simulink model "TCS0731"  (R2022b)
settings: Solver=VariableStepAuto  StartTime=0.0  StopTime=30  FixedStep=0.01  RelTol=1e-3
libraries: simulink x8, Solver_SF x1
settings Model: Creator=12045  LastModifiedBy=12045
settings DebuggingCC: ParameterPrecisionLossMsg=none

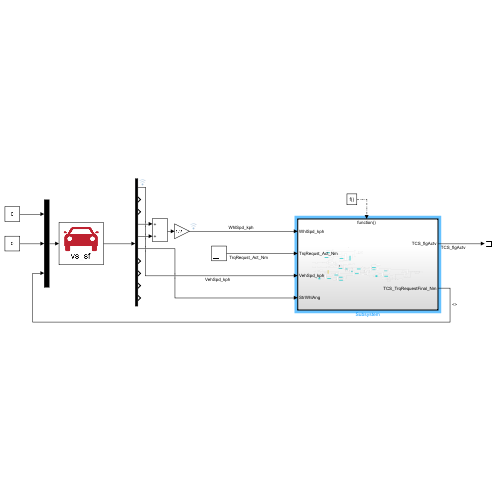
[thumbnail: Simulink's stored preview of the top-level diagram]
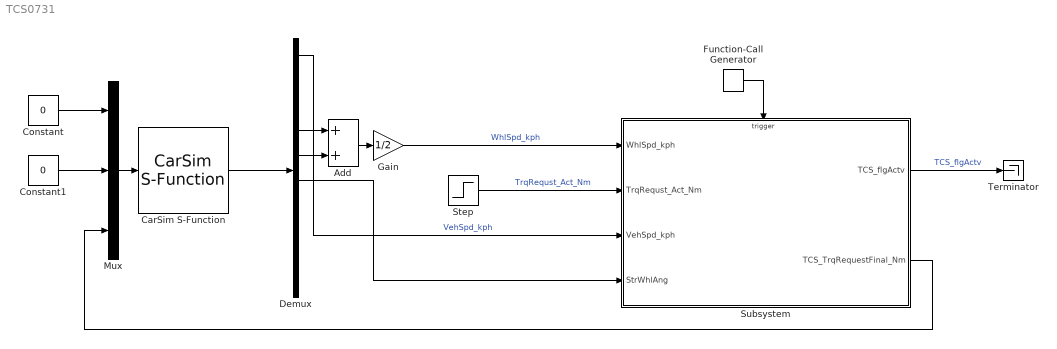
== system TCS0731 ==
  Add : Sum
  CarSim S-Function : Solver_SF/CarSim S-Function  Priority=1  SIMFILE=simfile.sim  Run_RTs=off  vs_state_ind=Run  StopMode_ind=Vehicle Model
  Constant : Constant  Value=0
  Constant1 : Constant  Value=0
  Demux : Demux  Outputs=10
  Function-Call Generator : simulink/Ports & Subsystems/Function-Call Generator  sample_time=0.01  numberOfIterations=1  DisallowWideOutput=off
  Gain : Gain  Gain=1/2
  Mux : Mux  Inputs=3
  Step : Step  After=80  SampleTime=0
  Subsystem : Subsystem
  Terminator : Terminator
  wires:
  Subsystem/1(TCS_flgActv) -> Terminator/1  "TCS_flgActv"
  Subsystem/2(TCS_TrqRequestFinal_Nm) -> Mux/3
  Function-Call Generator/1 -> Subsystem/Trigger
  Gain/1 -> Subsystem/1(WhlSpd_kph)  "WhlSpd_kph"
  Step/1 -> Subsystem/2(TrqRequst_Act_Nm)  "TrqRequst_Act_Nm"
  Demux/1 -> Subsystem/3(VehSpd_kph)  "VehSpd_kph"
  Mux/1 -> CarSim S-Function/1
  Constant/1 -> Mux/1
  Constant1/1 -> Mux/2
  CarSim S-Function/1 -> Demux/1
  Demux/4 -> Add/1
  Demux/5 -> Add/2
  Add/1 -> Gain/1
  Demux/6 -> Subsystem/4(StrWhlAng)

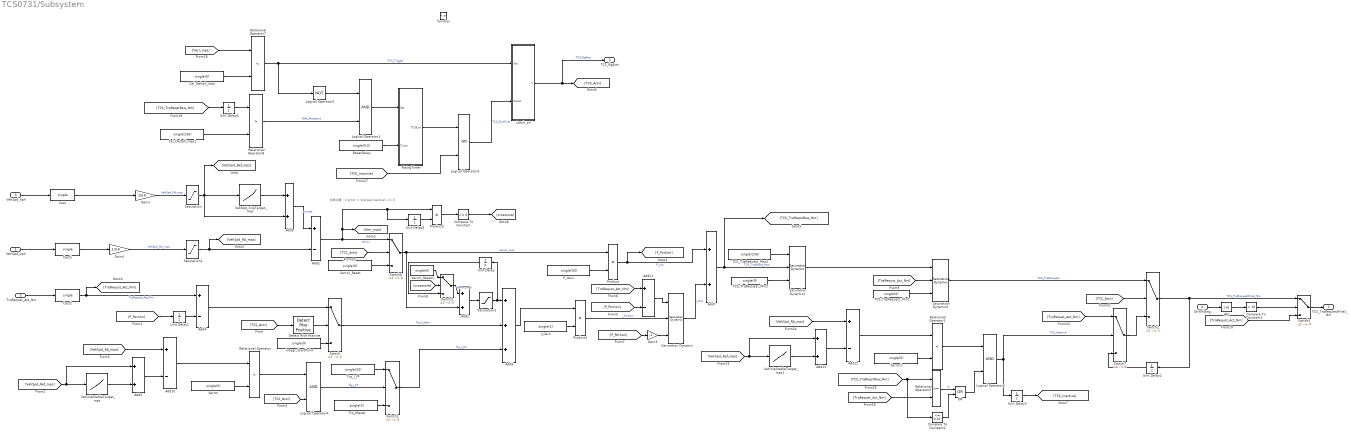
== system TCS0731/Subsystem ==
  note: 特殊设置：V error = Vtarget-Vactual <= 0
  WhlSpd_kph : Inport
  TrqRequst_Act_Nm : Inport  Port=2
  VehSpd_kph : Inport  Port=3
  StrWhlAng : Inport  Port=4
  function : TriggerPort  TriggerType=function-call  VariantControl=(inherit)
  Abs : Abs  SaturateOnIntegerOverflow=off
  Add{1,4,10..12} (5 alike) : Sum  Inputs=+-
  Add{2,5,7,9,13} (5 alike) : Sum
  Add6 : Sum  Inputs=+++
  Cal_DeltaV_mps : Constant  Value=single(0)
  Cal_DeltaV_mps1 : Constant  Value=single(235)
  Cast : DataTypeConversion  OutDataTypeStr=single  SaturateOnIntegerOverflow=off  RndMeth=Floor
  Cast1 : DataTypeConversion  OutDataTypeStr=single  SaturateOnIntegerOverflow=off  RndMeth=Floor
  Cast2 : DataTypeConversion  OutDataTypeStr=single  SaturateOnIntegerOverflow=off  RndMeth=Floor
  Compare To Constant : simulink/Logic and Bit Operations/Compare To Constant  relop=<=  const=0  OutDataTypeStr=boolean
  Compare To Constant1 : simulink/Logic and Bit Operations/Compare To Constant  relop=<  const=10  OutDataTypeStr=boolean
  Compare To Constant2 : simulink/Logic and Bit Operations/Compare To Constant  relop=<=  const=0.01  OutDataTypeStr=boolean
  Detect Rise Positive : simulink/Logic and Bit Operations/Detect Rise Positive  vinit=0  OutDataTypeStr=boolean
  Gain1 : Gain  Gain=1/3.6
  Gain3 : Gain  Gain=-1
  Gain4 : Gain  Gain=1/3.6
  I_Gain : Constant  Value=single(2)
  Integr_StartPoint : Constant  Value=single(0)
  Latch_on : Subsystem
  Logical Operator1 : Logic  AllPortsSameDT=off  OutDataTypeStr=boolean
  Logical Operator2 : Logic  Operator=NOT  AllPortsSameDT=off  OutDataTypeStr=boolean
  Logical Operator3 : Logic  Operator=OR  AllPortsSameDT=off  OutDataTypeStr=boolean
  Logical Operator4 : Logic  AllPortsSameDT=off  OutDataTypeStr=boolean
  Logical Operator5 : Logic  AllPortsSameDT=off  OutDataTypeStr=boolean
  OR : Logic  Operator=OR  AllPortsSameDT=off  OutDataTypeStr=boolean
  P_Gain : Constant  Value=single(20)
  Product : Product
  Product1 : Product
  Product2 : Product
  Relational Operator : RelationalOperator  Operator=<  OutDataTypeStr=boolean  RndMeth=Simplest  InputSameDT=off
  Relational Operator1 : RelationalOperator  Operator=<  OutDataTypeStr=boolean  RndMeth=Simplest  InputSameDT=off
  Relational Operator2 : RelationalOperator  OutDataTypeStr=boolean  RndMeth=Simplest  InputSameDT=off
  Relational Operator7 : RelationalOperator  Operator=<  OutDataTypeStr=boolean  RndMeth=Simplest  InputSameDT=off
  Relational Operator8 : RelationalOperator  Operator=>  OutDataTypeStr=boolean  RndMeth=Simplest  InputSameDT=off
  ResetDelay : Constant  Value=single(0.5)
  RisingTimer : Subsystem
  Saturation : Saturate  UpperLimit=40  LowerLimit=0
  Saturation Dynamic : simulink/Discontinuities/Saturation Dynamic  OutMin=[]  OutMax=[]  OutDataTypeStr=Inherit: Same as second input  OutDataType=fixdt(1, 16)  OutScaling=2^-10  DoSatur=off
  Saturation Dynamic1 : simulink/Discontinuities/Saturation Dynamic  OutMin=[]  OutMax=[]  OutDataTypeStr=Inherit: Same as second input  OutDataType=fixdt(1, 16)  OutScaling=2^-10  DoSatur=off
  Saturation Dynamic2 : simulink/Discontinuities/Saturation Dynamic  OutMin=[]  OutMax=[]  OutDataTypeStr=Inherit: Same as second input  OutDataType=fixdt(1, 16)  OutScaling=2^-10  DoSatur=off
  Saturation1 : Saturate  UpperLimit=50  LowerLimit=0
  Saturation2 : Saturate  UpperLimit=400  LowerLimit=-100
  Switch{,1..3,5..7} (7 alike) : Switch  Criteria=u2 ~= 0  SaturateOnIntegerOverflow=off  InputSameDT=off
  TCS_TrqRequest_Max2 : Constant  Value=single(235)
  TCS_TrqRequest_Min1 : Constant  Value=single(0)
  TCS_TrqRequest_Min2 : Constant  Value=single(0)
  Trq_IReset : Constant  Value=single(0)
  Trq_I_FF : Constant  Value=single(20)
  Unit Delay{,1..5} (6 alike) : UnitDelay  SampleTime=-1  HasFrameUpgradeWarning=on
  VehSpd_SlipTarget_mps : Lookup_n-D  NumberOfTableDimensions=1  BreakpointsForDimension1=[0 3 25 30]  Table=[0.3,0.3,2.5,2.5]  ExtrapMethod=Clip  InternalRulePriority=Speed  RndMeth=Simplest
  VehicleStableTarget_mps : Lookup_n-D  NumberOfTableDimensions=1  BreakpointsForDimension1=[0,3,25,30]  Table=[0.4,0.4,1.2,1.2]  ExtrapMethod=Clip  InternalRulePriority=Speed  RndMeth=Simplest
  VehicleStableTarget_mps1 : Lookup_n-D  NumberOfTableDimensions=1  BreakpointsForDimension1=[0,3,25,30]  Table=[0.2,0.2,1.2,1.2]  ExtrapMethod=Clip  InternalRulePriority=Speed  RndMeth=Simplest
  Verror : Constant  Value=single(0)
  Verror1 : Constant  Value=single(0)
  Verror_Reset : Constant  Value=single(0)
  Verror_Reset1 : Constant  Value=single(0)
  TCS_flgActv : Outport
  TCS_TrqRequestFinal_Nm : Outport  Port=2
  wires:
  TCS_TrqRequest_Max2/1 -> Saturation Dynamic1/1
  [TCS_Actv] -> Switch2/2
  [TrqRequst_Act_Nm] -> Switch7/1
  [VehSpd_Ref_mps] -> VehicleStableTarget_mps1/1, Add13/1
  Integr_StartPoint/1 -> Switch/3
  VehicleStableTarget_mps1/1 -> Add13/2
  [VehSpd_Ref_mps] -> Add5/1, VehicleStableTarget_mps/1
  [VehSpd_RA_mps] -> Add12/1
  [TCS_Actv] -> Switch6/2
  Gain4/1 -> Saturation1/1  "VehSpd_RA_mps"
  [TCS_Actv] -> Detect Rise Positive/1
  Saturation Dynamic1/1 -> Saturation Dynamic2/1
  Logical Operator3/1 -> Latch_on/2(Reset)  "TCS_ExitFinal"
  ResetDelay/1 -> RisingTimer/2(Timer)
  Latch_on/1(flg_TCSActv) -> TCS_flgActv/1, [TCS_Actv]  "TCS_flgActv"
  Unit Delay4/1 -> Relational Operator8/1
  WhlSpd_kph/1 -> Cast1/1
  Relational Operator1/1 -> Logical Operator5/1
  Product/1 -> [P_Portion], Add7/1  "P_out"
  Relational Operator7/1 -> Latch_on/1(Set), Logical Operator2/1  "TCS_Trigger"
  Switch/1 -> Add6/2  "Trq_I_Start"
  Trq_I_FF/1 -> Switch1/1
  Add13/1 -> Add12/2
  [TrqRequst_Act_Nm] -> Relational Operator2/2
  Add2/1 -> Saturation2/1
  TCS_TrqRequest_Min2/1 -> Saturation Dynamic1/3
  Add4/1 -> Switch/1
  [TCS_Inactive] -> Logical Operator3/2
  Add10/1 -> Relational Operator/1
  VehicleStableTarget_mps/1 -> Add5/2
  TrqRequst_Act_Nm/1 -> Cast2/1
  [P_Portion] -> Gain3/1
  Gain1/1 -> Saturation/1  "VehSpd_FA_mps"
  Saturation1/1 -> Add1/2, [VehSpd_RA_mps]
  Product1/1 -> Saturation Dynamic/2  "I_Portion"
  Logical Operator5/1 -> Unit Delay3/1, Switch7/2  "TCS_Inactive"
  Cal_DeltaV_mps1/1 -> Relational Operator8/2
  Add11/1 -> Saturation Dynamic/1
  Unit Delay3/1 -> [TCS_Inactive]
  Logical Operator1/1 -> RisingTimer/1(Set)
  [P_Portion] -> Add11/2
  Switch2/1 -> Switch5/1, Unit Delay2/1  "TCS_TrqRequestFinal_Nm"
  [TCS_TrqReqstRaw_Nm] -> Compare To Constant2/1, Relational Operator2/1
  Switch1/1 -> Add6/3  "Trq_I_FF"
  [VehSpd_RA_mps] -> Add10/1
  Unit Delay/1 -> Switch3/3
  Logical Operator2/1 -> Logical Operator1/1
  Trq_IReset/1 -> Switch1/3
  Verror1/1 -> Relational Operator1/2
  Relational Operator2/1 -> OR/1  "a"
  Switch7/1 -> Switch2/3
  Add12/1 -> Relational Operator1/1
  [P_Portion] -> Unit Delay1/1
  Unit Delay1/1 -> Add4/2
  Verror/1 -> Relational Operator/2
  Saturation Dynamic2/1 -> Switch2/1  "TCS_TrqRequest"
  [TrqRequst_Act_Nm] -> Saturation Dynamic2/2
  [TrqRequst_Act_Nm] -> Add11/1
  I_Gain/1 -> Product1/2
  Switch6/1 -> Product/1, Add2/2  "Verror_mps"
  Add9/1 -> Add1/1  "whlref"
  VehSpd_SlipTarget_mps/1 -> Add9/1
  [TCS_TrqReqstRaw_Nm] -> Unit Delay4/1
  Add5/1 -> Add10/2
  Saturation2/1 -> Unit Delay/1, Add6/1
  Add1/1 -> Switch6/1, [Verr_mps], Unit Delay5/1, Product2/1  "Verror"
  Verror_Reset/1 -> Switch6/3
  TCS_TrqRequest_Min1/1 -> Saturation Dynamic2/3
  Add7/1 -> Saturation Dynamic1/2, [TCS_TrqReqstRaw_Nm]  "TCS_TrqReqst_Raw"
  [Verr_mps] -> Relational Operator7/1
  Cal_DeltaV_mps/1 -> Relational Operator7/2
  Add6/1 -> Product1/1
  Relational Operator8/1 -> Logical Operator1/2  "fSat_Actuators"
  Relational Operator/1 -> Logical Operator4/1
  Saturation/1 -> Add9/2, VehSpd_SlipTarget_mps/1, [VehSpd_Ref_mps]
  P_Gain/1 -> Product/2
  Detect Rise Positive/1 -> Switch/2
  [TCS_Actv] -> Logical Operator4/2
  Gain3/1 -> Saturation Dynamic/3
  Logical Operator4/1 -> Switch1/2  "flg_I_FF"
  VehSpd_kph/1 -> Cast/1
  RisingTimer/1(TCSExit) -> Logical Operator3/1
  Saturation Dynamic/1 -> Add7/2  "I_Out"
  Cast/1 -> Gain1/1
  Cast1/1 -> Gain4/1
  Cast2/1 -> Add4/1, [TrqRequst_Act_Nm]  "TrqRequst_Act_Nm"
  Unit Delay5/1 -> Product2/2
  Product2/1 -> Compare To Constant/1
  Switch3/1 -> Add2/1  "Verror_mps"
  Compare To Constant/1 -> [crosszore]
  [crosszore] -> Switch3/2
  Verror_Reset1/1 -> Switch3/1
  StrWhlAng/1 -> Abs/1
  Abs/1 -> Compare To Constant1/1
  Compare To Constant1/1 -> Switch5/2
  [TrqRequst_Act_Nm] -> Switch5/3
  Unit Delay2/1 -> Switch7/3
  Switch5/1 -> TCS_TrqRequestFinal_Nm/1
  Compare To Constant2/1 -> OR/2
  OR/1 -> Logical Operator5/2

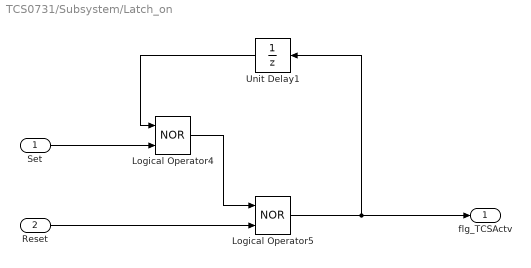
== system TCS0731/Subsystem/Latch_on ==
  Set : Inport
  Reset : Inport  Port=2
  Logical Operator4 : Logic  Operator=NOR  AllPortsSameDT=off  OutDataTypeStr=boolean
  Logical Operator5 : Logic  Operator=NOR  AllPortsSameDT=off  OutDataTypeStr=boolean
  Unit Delay1 : UnitDelay  SampleTime=-1  HasFrameUpgradeWarning=on
  flg_TCSActv : Outport
  wires:
  Logical Operator5/1 -> flg_TCSActv/1, Unit Delay1/1
  Reset/1 -> Logical Operator5/2
  Unit Delay1/1 -> Logical Operator4/1
  Set/1 -> Logical Operator4/2
  Logical Operator4/1 -> Logical Operator5/1

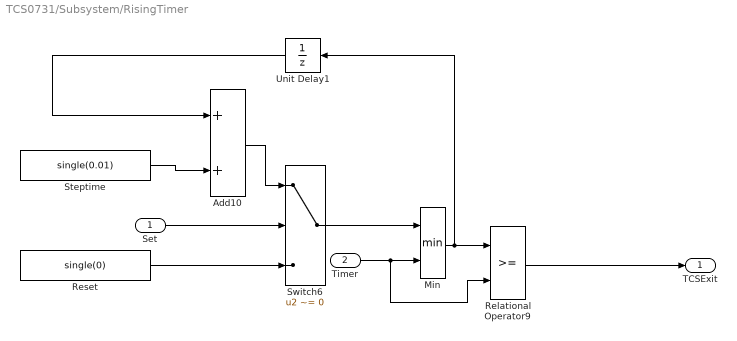
== system TCS0731/Subsystem/RisingTimer ==
  Set : Inport
  Timer : Inport  Port=2
  Add10 : Sum
  Min : MinMax  Inputs=2
  Relational Operator9 : RelationalOperator  OutDataTypeStr=boolean  RndMeth=Simplest  InputSameDT=off
  Reset : Constant  Value=single(0)
  Steptime : Constant  Value=single(0.01)
  Switch6 : Switch  Criteria=u2 ~= 0  SaturateOnIntegerOverflow=off  InputSameDT=off
  Unit Delay1 : UnitDelay  SampleTime=-1  HasFrameUpgradeWarning=on
  TCSExit : Outport
  wires:
  Add10/1 -> Switch6/1
  Set/1 -> Switch6/2
  Min/1 -> Unit Delay1/1, Relational Operator9/1
  Unit Delay1/1 -> Add10/1
  Timer/1 -> Relational Operator9/2, Min/2
  Reset/1 -> Switch6/3
  Relational Operator9/1 -> TCSExit/1
  Steptime/1 -> Add10/2
  Switch6/1 -> Min/1
